simulink model "test_x_eng_sim_packet_4a"  (Simulink 6.2)
settings: Solver=ode45  StartTime=0.0  StopTime=600000  RelTol=1e-3
undefined symbols (not defined in the file or in its folder): ant_bits, BitWidth, cmult_4bit_em
libraries: xbsIndex_r3 x798, casper_library x39, xps_library x27, simulink x1
(part 1 of 6)
settings Model: LastModifiedBy=dsp
settings DebuggingCC: SolverPrmCheckMsg=warning

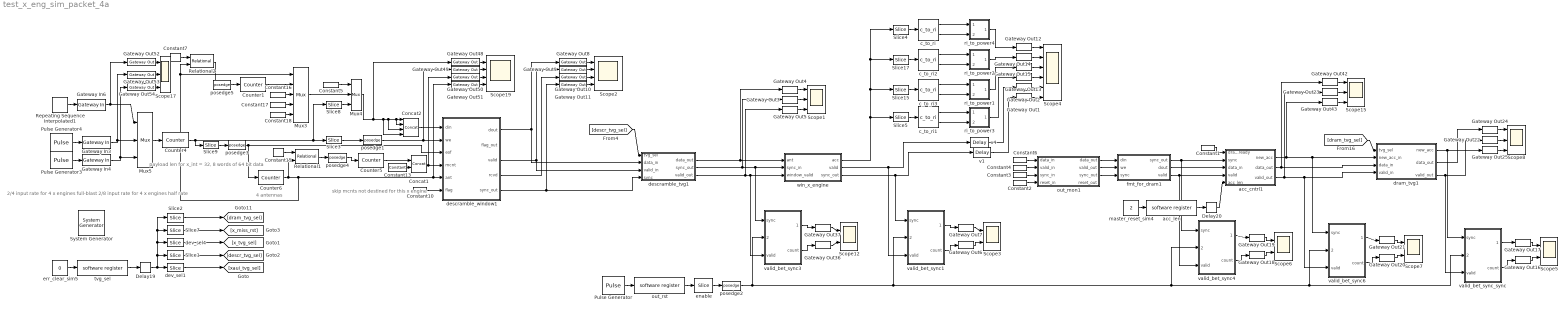
== system test_x_eng_sim_packet_4a ==
  note: 2/4 input rate for 4 x engines full-blast
      | 2/8 input rate for 4 x engines half rate
  note: 4 antennas
  note: skip mcnts not destined
      | for this x engine
  note: payload len
      | for x_int = 32,
      | 8 words of 64 bit data
  " System Generator" : xbsIndex_r3/ System Generator  Tag=genX  xilinxfamily=Virtex2  part=xc2v1000  speed=-4  package=bg575  synthesis_tool=XST  directory=./netlist  testbench=off  simulink_period=1  sysclk_period=100  incr_netlist=off  trim_vbits=Everywhere in SubSystem  dbl_ovrd=According to Block Masks  core_generation=According to Block Masks  run_coregen=off  deprecated_control=off  eval_field=0
      settings: AttributesFormatString=System\nGenerator
  Concat1 : xbsIndex_r3/Concat  num_inputs=2  explicit_period=off  period=1  dbl_ovrd=off
  Concat2 : xbsIndex_r3/Concat  num_inputs=4  explicit_period=off  period=1  dbl_ovrd=off
  Constant1 : xbsIndex_r3/Constant  const=1  equ=P=C  arith_type=Boolean  n_bits=1  bin_pt=0  opselect=C  inp2=PCIN>>17  opr=+  inp1=P  carry=CIN  iostate=0  explicit_period=on  period=1  dbl_ovrd=off
  Constant10 : xbsIndex_r3/Constant  const=0  equ=P=C  arith_type=Unsigned  n_bits=1  bin_pt=0  opselect=C  inp2=PCIN>>17  opr=+  inp1=P  carry=CIN  iostate=0  explicit_period=on  period=1  dbl_ovrd=off
  Constant13 : xbsIndex_r3/Constant  const=0  equ=P=C  arith_type=Unsigned  n_bits=2  bin_pt=0  opselect=C  inp2=PCIN>>17  opr=+  inp1=P  carry=CIN  iostate=0  explicit_period=on  period=1  dbl_ovrd=off
  Constant15 : xbsIndex_r3/Constant  const=0  equ=P=C  arith_type=Unsigned  n_bits=3  bin_pt=0  opselect=C  inp2=PCIN>>17  opr=+  inp1=P  carry=CIN  iostate=0  explicit_period=on  period=1  dbl_ovrd=off
  Constant16 : xbsIndex_r3/Constant  const=0  equ=P=C  arith_type=Unsigned  n_bits=16  bin_pt=0  opselect=C  inp2=PCIN>>17  opr=+  inp1=P  carry=CIN  iostate=0  explicit_period=on  period=1  dbl_ovrd=off
  Constant17 : xbsIndex_r3/Constant  const=0  equ=P=C  arith_type=Unsigned  n_bits=16  bin_pt=0  opselect=C  inp2=PCIN>>17  opr=+  inp1=P  carry=CIN  iostate=0  explicit_period=on  period=1  dbl_ovrd=off
  Constant18 : xbsIndex_r3/Constant  const=0  equ=P=C  arith_type=Unsigned  n_bits=16  bin_pt=0  opselect=C  inp2=PCIN>>17  opr=+  inp1=P  carry=CIN  iostate=0  explicit_period=on  period=1  dbl_ovrd=off
  Constant2 : xbsIndex_r3/Constant  const=0  equ=P=C  arith_type=Boolean  n_bits=1  bin_pt=0  opselect=C  inp2=PCIN>>17  opr=+  inp1=P  carry=CIN  iostate=0  explicit_period=on  period=1  dbl_ovrd=off
  Constant3 : xbsIndex_r3/Constant  const=0  equ=P=C  arith_type=Boolean  n_bits=1  bin_pt=0  opselect=C  inp2=PCIN>>17  opr=+  inp1=P  carry=CIN  iostate=0  explicit_period=on  period=1  dbl_ovrd=off
  Constant4 : xbsIndex_r3/Constant  const=0  equ=P=C  arith_type=Boolean  n_bits=1  bin_pt=0  opselect=C  inp2=PCIN>>17  opr=+  inp1=P  carry=CIN  iostate=0  explicit_period=on  period=1  dbl_ovrd=off
  Constant5 : xbsIndex_r3/Constant  const=0  equ=P=C  arith_type=Unsigned  n_bits=1  bin_pt=0  opselect=C  inp2=PCIN>>17  opr=+  inp1=P  carry=CIN  iostate=0  explicit_period=on  period=1  dbl_ovrd=off
  Constant6 : xbsIndex_r3/Constant  const=0  equ=P=C  arith_type=Unsigned  n_bits=112  bin_pt=0  opselect=C  inp2=PCIN>>17  opr=+  inp1=P  carry=CIN  iostate=0  explicit_period=on  period=1  dbl_ovrd=off
  Constant7 : xbsIndex_r3/Constant  const=0  equ=P=C  arith_type=Unsigned  n_bits=1  bin_pt=0  opselect=C  inp2=PCIN>>17  opr=+  inp1=P  carry=CIN  iostate=0  explicit_period=on  period=1  dbl_ovrd=off
  Counter1 : xbsIndex_r3/Counter  cnt_type=Free Running  n_bits=16  bin_pt=0  arith_type=Unsigned  start_count=0  cnt_to=Inf  cnt_by_val=1  operation=Up  explicit_period=off  period=1  load_pin=off  rst=off  en=on  dbl_ovrd=off  show_param=off  use_rpm=on  gen_core=off
      settings: xl_area=[0, 0, 0, 0, 0, 0, 0]
  Counter4 : xbsIndex_r3/Counter  cnt_type=Free Running  n_bits=32  bin_pt=0  arith_type=Unsigned  start_count=0  cnt_to=32  cnt_by_val=1  operation=Up  explicit_period=off  period=1  load_pin=off  rst=off  en=on  dbl_ovrd=off  show_param=off  use_rpm=on  gen_core=off
      settings: xl_area=[0, 0, 0, 0, 0, 0, 0]
  Counter5 : xbsIndex_r3/Counter  cnt_type=Free Running  n_bits=48-2  bin_pt=0  arith_type=Unsigned  start_count=0  cnt_to=Inf  cnt_by_val=1  operation=Up  explicit_period=off  period=1  load_pin=off  rst=off  en=on  dbl_ovrd=off  show_param=off  use_rpm=on  gen_core=off
      settings: xl_area=[0, 0, 0, 0, 0, 0, 0]
  Counter6 : xbsIndex_r3/Counter  cnt_type=Free Running  n_bits=2  bin_pt=0  arith_type=Unsigned  start_count=0  cnt_to=Inf  cnt_by_val=1  operation=Up  explicit_period=off  period=1  load_pin=off  rst=off  en=on  dbl_ovrd=off  show_param=off  use_rpm=on  gen_core=off
      settings: xl_area=[0, 0, 0, 0, 0, 0, 0]
  Delay19 : xbsIndex_r3/Delay  latency=2  reg_retiming=off  explicit_period=off  period=1  en=off  accept_only_valid=off  init_zero=on  dbl_ovrd=off  show_param=off
      settings: xl_area=[0, 0, 0, 0, 0, 0, 0]
  Delay20 : xbsIndex_r3/Delay  latency=2  reg_retiming=off  explicit_period=off  period=1  en=off  accept_only_valid=off  init_zero=on  dbl_ovrd=off  show_param=off
      settings: xl_area=[0, 0, 0, 0, 0, 0, 0]
  Gateway In3 : xbsIndex_r3/Gateway In  arith_type=Boolean  n_bits=8  bin_pt=6  quantization=Truncate  overflow=Wrap  period=1  timing_constraint=None  locs_specified=off  LOCs={}  needs_fixed_name=off  dbl_ovrd=off  show_param=off
      settings: xl_area=[0, 0, 0, 0, 0, 0, 0]
  Gateway In4 : xbsIndex_r3/Gateway In  arith_type=Boolean  n_bits=8  bin_pt=6  quantization=Truncate  overflow=Wrap  period=1  timing_constraint=None  locs_specified=off  LOCs={}  needs_fixed_name=off  dbl_ovrd=off  show_param=off
      settings: xl_area=[0, 0, 0, 0, 0, 0, 0]
  Gateway In6 : xbsIndex_r3/Gateway In  arith_type=Unsigned  n_bits=1  bin_pt=0  quantization=Truncate  overflow=Wrap  period=1  timing_constraint=None  locs_specified=off  LOCs={}  needs_fixed_name=off  dbl_ovrd=off  show_param=off
      settings: xl_area=[0, 0, 0, 0, 0, 0, 0]
  Gateway Out{1..7,12..25,36..37,42..43} (25 alike) : xbsIndex_r3/Gateway Out  output_type=Double  nbits=8  bin_pt=6  arith_type=Boolean  quantization=Truncate  overflow=Wrap  hdl_port=off  timing_constraint=None  locs_specified=off  LOCs={}  needs_fixed_name=off  show_param=off
      settings: xl_area=[0, 0, 0, 0, 0, 0, 0]
  Gateway Out{8..11,48..54} (11 alike) : xbsIndex_r3/Gateway Out  output_type=Double  nbits=8  bin_pt=6  arith_type=Boolean  quantization=Truncate  overflow=Wrap  hdl_port=on  timing_constraint=None  locs_specified=off  LOCs={}  needs_fixed_name=off  show_param=off
      settings: xl_area=[0, 0, 0, 0, 0, 0, 0]
  Mux3 : xbsIndex_r3/Mux  inputs=4  precision=Full  arith_type="Signed  (2's comp)"  n_bits=8  bin_pt=2  quantization=Truncate  overflow=Wrap  latency=0  explicit_period=off  period=1  en=off  dbl_ovrd=off  show_param=off  mux_type=off  use_rpm=off  gen_core=off
      settings: xl_area=[0, 0, 0, 0, 0, 0, 0]
  Mux4 : xbsIndex_r3/Mux  inputs=2  precision=Full  arith_type="Signed  (2's comp)"  n_bits=8  bin_pt=2  quantization=Truncate  overflow=Wrap  latency=0  explicit_period=off  period=1  en=off  dbl_ovrd=off  show_param=off  mux_type=off  use_rpm=off  gen_core=off
      settings: xl_area=[0, 0, 0, 0, 0, 0, 0]
  Mux5 : xbsIndex_r3/Mux  inputs=2  precision=Full  arith_type="Signed  (2's comp)"  n_bits=8  bin_pt=2  quantization=Truncate  overflow=Wrap  latency=0  explicit_period=off  period=1  en=off  dbl_ovrd=off  show_param=off  mux_type=off  use_rpm=off  gen_core=off
      settings: xl_area=[0, 0, 0, 0, 0, 0, 0]
  Pulse Generator : DiscretePulseGenerator  Period=2^15  PhaseDelay=2^14
  Pulse Generator3 : DiscretePulseGenerator  Period=4  PulseWidth=2
  Pulse Generator4 : DiscretePulseGenerator  PulseWidth=2
  Relational1 : xbsIndex_r3/Relational  mode=a=b  latency=1  explicit_period=off  period=1  en=off  dbl_ovrd=off  show_param=off
      settings: xl_area=[0, 0, 0, 0, 0, 0, 0]
  Relational2 : xbsIndex_r3/Relational  mode=a=b  latency=1  explicit_period=off  period=1  en=off  dbl_ovrd=off  show_param=off
      settings: xl_area=[0, 0, 0, 0, 0, 0, 0]
  Repeating Sequence Interpolated1 : simulink/Sources/Repeating Sequence Interpolated  OutValues=[0 1].'  TimeValues=[100000 300000].'  LookUpMeth=Use Input Above  tsamp=1  OutputDataTypeScalingMode=Specify via dialog  OutDataType=float('double')  OutScaling=2^-10
  Scope{1,8,15,17} (4 alike) : Scope  NumInputPorts=3
      Scope1 settings: YMin=-1~-1~-5  YMax=1~1~5  SaveName=ScopeData5
      Scope15 settings: YMin=0~0~-1  YMax=1.4e+011~1~1  SaveName=ScopeData12
      Scope17 settings: YMin=-1~0~0  YMax=1~1~1  SaveName=ScopeData9
      Scope8 settings: YMin=0~0~-1  YMax=1.1e+011~1~1  SaveName=ScopeData10
  Scope{3,5..7,12} (5 alike) : Scope  NumInputPorts=2
      Scope12 settings: YMin=31128.7~9840  YMax=34405.3~10060  SaveName=data_into_xeng
      Scope3 settings: YMin=2560~1140  YMax=2560~1150  SaveName=data_into_xeng1
      Scope5 settings: YMin=9727.05~819  YMax=10751~839  SaveName=ScopeData6
      Scope6 settings: YMin=4864~2340  YMax=5376~2360  SaveName=ScopeData4
      Scope7 settings: YMin=0~0  YMax=10500~10500  SaveName=ScopeData8
  Scope19 : Scope  NumInputPorts=4
      settings: YMin=0~0~28~0  YMax=1~1~40~3  SaveName=ScopeData14
  Scope2 : Scope  NumInputPorts=4
      settings: YMin=0~1~1~0  YMax=32.5~1~1~1
  Scope4 : Scope  NumInputPorts=6
      settings: YMin=-1~0~-1~-1~0~-1  YMax=1~4~1~1~1~1  SaveName=ScopeData7
  Slice1 : xbsIndex_r3/Slice  mode=Lower Bit Location + Width  nbits=2  bit1=0  base1=MSB of Input  bit0=1  base0=LSB of Input  boolean_output=on  explicit_period=off  period=1  dbl_ovrd=off
  Slice15 : xbsIndex_r3/Slice  mode=Lower Bit Location + Width  nbits=112/4  bit1=0  base1=MSB of Input  bit0=112/4  base0=LSB of Input  boolean_output=off  explicit_period=off  period=1  dbl_ovrd=off
  Slice17 : xbsIndex_r3/Slice  mode=Lower Bit Location + Width  nbits=112/4  bit1=0  base1=MSB of Input  bit0=112/4*2  base0=LSB of Input  boolean_output=off  explicit_period=off  period=1  dbl_ovrd=off
  Slice2 : xbsIndex_r3/Slice  mode=Lower Bit Location + Width  nbits=5  bit1=0  base1=MSB of Input  bit0=9  base0=LSB of Input  boolean_output=off  explicit_period=off  period=1  dbl_ovrd=off
  Slice3 : xbsIndex_r3/Slice  mode=Lower Bit Location + Width  nbits=1  bit1=0  base1=MSB of Input  bit0=0  base0=LSB of Input  boolean_output=on  explicit_period=off  period=1  dbl_ovrd=off
  Slice4 : xbsIndex_r3/Slice  mode=Lower Bit Location + Width  nbits=112/4  bit1=0  base1=MSB of Input  bit0=112/4*3  base0=LSB of Input  boolean_output=off  explicit_period=off  period=1  dbl_ovrd=off
  Slice5 : xbsIndex_r3/Slice  mode=Lower Bit Location + Width  nbits=112/4  bit1=0  base1=MSB of Input  bit0=0  base0=LSB of Input  boolean_output=off  explicit_period=off  period=1  dbl_ovrd=off
  Slice7 : xbsIndex_r3/Slice  mode=Lower Bit Location + Width  nbits=1  bit1=0  base1=MSB of Input  bit0=8  base0=LSB of Input  boolean_output=on  explicit_period=off  period=1  dbl_ovrd=off
  Slice8 : xbsIndex_r3/Slice  mode=Lower Bit Location + Width  nbits=16  bit1=0  base1=MSB of Input  bit0=1  base0=LSB of Input  boolean_output=on  explicit_period=off  period=1  dbl_ovrd=off
  Slice9 : xbsIndex_r3/Slice  mode=Lower Bit Location + Width  nbits=1  bit1=0  base1=MSB of Input  bit0=4  base0=LSB of Input  boolean_output=on  explicit_period=off  period=1  dbl_ovrd=off
  acc_cntrl1 : Subsystem
  acc_len : xps_library/software register  Tag=xps:sw_reg  io_dir=From Processor  arith_type=Unsigned  bitwidth=32  bin_pt=0  sample_period=1  gw_name=test_x_eng_sim_packet_4a_acc_len_user_data_out
  c_to_ri{,1..3} (4 alike) : casper_library/Misc/c_to_ri  n_bits=16  bin_pt=6
      settings: AttributesFormatString=16_6 r/i
  descramble_tvg1 : Subsystem  mask{ant_bits=2, x_int_bits=5, sync_period=15}
      mask prompts: ant_bits "Number of Antennas (2^?):"; x_int_bits "X Integration Length (2^?):"; sync_period "Sync Pulse Period (2^?):"
  descramble_window1 : Subsystem  mask{ant_bits=2, x_int_bits=5, window_bits=3, sync_bits=11}
      mask prompts: ant_bits "Maximum Number of Antennas (2^?):"; x_int_bits "X Engine Integration Length (2^?):"; window_bits "Number of Windows to Buffer (2^?):"; sync_bits "Samples Between Sync Pulses (2^?)"
      mask help: Valids between sync pulses: Would like this to come after every dram_vecc_len: valids_bet_syncs = xeng_int_len * num_ants * freqs_per_xeng. Normally, num_ants = num_xeng so this simplifies to xeng_int_len * n_chans.
  dev_sel1 : xbsIndex_r3/Slice  mode=Lower Bit Location + Width  nbits=1  bit1=0  base1=MSB of Input  bit0=0  base0=LSB of Input  boolean_output=off  explicit_period=off  period=1  dbl_ovrd=off
  dev_sel4 : xbsIndex_r3/Slice  mode=Lower Bit Location + Width  nbits=2  bit1=0  base1=MSB of Input  bit0=3  base0=LSB of Input  boolean_output=off  explicit_period=off  period=1  dbl_ovrd=off
  dram_tvg1 : Subsystem  mask{len=18432}
      mask prompts: len "Number of Vectors"
  enable : xbsIndex_r3/Slice  mode=Lower Bit Location + Width  nbits=1  bit1=0  base1=LSB of Input  bit0=0  base0=LSB of Input  boolean_output=on  explicit_period=off  period=1  dbl_ovrd=off
  err_clear_sim5 : Constant  Value=0
  fmt_for_dram1 : Subsystem  mask{x_int_bits=5, x_n_bits=4}
      mask prompts: x_int_bits "X Engine integration length (2^?):"; x_n_bits "X Engine input bits"
  master_reset_sim4 : Constant  Value=2
  out_mon1 : Subsystem  mask{n_ants=4, n_chans=512}
      mask prompts: n_ants "Number of Antennas"; n_chans "Number of Frequency Channels in the system"
  out_rst : xps_library/software register  Tag=xps:sw_reg  io_dir=From Processor  arith_type=Unsigned  bitwidth=32  bin_pt=0  sample_period=1  gw_name=test_x_eng_sim_packet_4a_out_rst_user_data_out
  posedge{1..5} (5 alike) : casper_library/Misc/posedge  Tag=Rising Edge Detector
  ri_to_power1 : Subsystem
  ri_to_power2 : Subsystem
  ri_to_power3 : Subsystem
  ri_to_power4 : Subsystem
  tvg_sel : xps_library/software register  Tag=xps:sw_reg  io_dir=From Processor  arith_type=Unsigned  bitwidth=32  bin_pt=0  sample_period=1  gw_name=test_x_eng_sim_packet_4a_tvg_sel_user_data_out
  v1 : xbsIndex_r3/Delay  latency=5  reg_retiming=off  explicit_period=off  period=1  en=off  accept_only_valid=off  init_zero=on  dbl_ovrd=off  show_param=off
      settings: xl_area=[0, 0, 0, 0, 0, 0, 0]
  v4 : xbsIndex_r3/Delay  latency=5  reg_retiming=off  explicit_period=off  period=1  en=off  accept_only_valid=off  init_zero=on  dbl_ovrd=off  show_param=off
      settings: xl_area=[0, 0, 0, 0, 0, 0, 0]
  valid_bet_sync1 : Subsystem
  valid_bet_sync3 : Subsystem
  valid_bet_sync4 : Subsystem
  valid_bet_sync6 : Subsystem
  valid_bet_sync_sync : Subsystem
  win_x_engine : Subsystem  AncestorBlock=casper_library/Correlator/x_engine  mask(x_engine){n_ants=4, n_bits=4, acc_len=32, add_latency=1, mult_latency=1, bram_latency=1, use_ded_mult=1, use_bram_delay=1}
      mask prompts: n_ants "Number of Antennas"; n_bits "Bit Width of Samples In"; acc_len "Accumulation Length"; add_latency "Add Latency"; mult_latency "Mult Latency"; bram_latency "BRAM Latency"; use_ded_mult "Multiplier Type (0=slices 1=embedded 2=bram)"; use_bram_delay "Delay in BRAM"
      mask init:
      | bit_growth = ceil(log2(acc_len));
      | ant_bits = ceil(log2(n_ants));
      | n_bits_out = (2*n_bits + 1 + bit_growth);
      | 
      | win_x_engine_init(gcb, ...
      |     'n_ants', n_ants, ...
      |     'n_bits', n_bits, ...
      |     'acc_len', acc_len, ...
      |     'add_latency', add_latency, ...
      |     'mult_latency', mult_latency, ...
      |     'bram_latency', bram_latency, ...
      |     'use_ded_mult', use_ded_mult, ...
      |     'use_bram_delay', use_bram_delay);
      settings: AttributesFormatString=n_ant=4, bits=4, mult=1, bram=1
  wires:
  [descr_tvg_sel] -> descramble_tvg1/1(tvg_sel)
  descramble_tvg1/1(data_out) -> win_x_engine/1(ant), Gateway Out4/1
  out_rst/1 -> enable/1
  Pulse Generator/1 -> out_rst/1
  enable/1 -> posedge2/1
  posedge2/1 -> valid_bet_sync3/2(rst_max), valid_bet_sync1/2(rst_max), valid_bet_sync4/2(rst_max), valid_bet_sync6/2(rst_max), valid_bet_sync_sync/2(rst_max)
  Gateway Out8/1 -> Scope2/1
  Gateway Out9/1 -> Scope2/2
  Gateway Out10/1 -> Scope2/3
  Gateway Out11/1 -> Scope2/4
  err_clear_sim5/1 -> tvg_sel/1
  tvg_sel/1 -> Delay19/1
  Delay19/1 -> dev_sel1/1, Slice1/1, dev_sel4/1, Slice2/1, Slice7/1
  dev_sel1/1 -> [xaui_tvg_sel]
  Slice1/1 -> [descr_tvg_sel]
  dev_sel4/1 -> [x_tvg_sel]
  Slice7/1 -> [x_miss_rst]
  Slice2/1 -> [dram_tvg_sel]
  Gateway Out36/1 -> Scope12/2
  Gateway Out37/1 -> Scope12/1
  valid_bet_sync3/1(max_count) -> Gateway Out37/1
  valid_bet_sync3/2(count) -> Gateway Out36/1
  Constant10/1 -> descramble_window1/6(flag)
  Gateway Out48/1 -> Scope19/1
  Gateway Out49/1 -> Scope19/2
  Gateway Out50/1 -> Scope19/3
  Gateway Out51/1 -> Scope19/4
  Constant13/1 -> Concat1/2
  Concat1/1 -> Gateway Out50/1, descramble_window1/4(mcnt)
  Counter5/1 -> Concat1/1
  Counter6/1 -> Relational1/2, Gateway Out51/1, descramble_window1/5(ant), Mux3/1, Relational2/2
  Concat2/1 -> descramble_window1/1(din)
  Relational1/1 -> posedge4/1
  Constant15/1 -> Relational1/1
  Slice3/1 -> posedge1/1
  Counter4/1 -> Slice9/1, Slice3/1, Slice8/1
  Mux4/1 -> Concat2/4, Concat2/3, Concat2/1, Concat2/2, Gateway Out48/1
  Slice9/1 -> posedge3/1
  posedge3/1 -> Counter6/1, descramble_window1/3(eof)
  posedge4/1 -> Counter5/1
  Pulse Generator3/1 -> Gateway In4/1
  Counter1/1 -> Mux3/2
  Constant16/1 -> Mux3/3
  Constant17/1 -> Mux3/4
  Constant18/1 -> Mux3/5
  Mux3/1 -> Mux4/2
  Slice8/1 -> Mux4/3
  Constant5/1 -> Mux4/1
  Pulse Generator4/1 -> Gateway In3/1
  Mux5/1 -> Counter4/1
  Gateway In3/1 -> Gateway Out53/1, Mux5/2
  Gateway In4/1 -> Gateway Out54/1, Mux5/3
  Gateway In6/1 -> Mux5/1, Gateway Out52/1
  Repeating Sequence Interpolated1/1 -> Gateway In6/1
  Gateway Out52/1 -> Scope17/1
  Gateway Out53/1 -> Scope17/2
  Gateway Out54/1 -> Scope17/3
  descramble_tvg1/3(valid_out) -> valid_bet_sync3/3(valid), win_x_engine/3(window_valid), Gateway Out5/1
  posedge1/1 -> Gateway Out49/1, descramble_window1/2(we)
  win_x_engine/1(acc) -> Slice4/1, Slice17/1, Slice15/1, Slice5/1
  win_x_engine/2(valid) -> valid_bet_sync1/3(valid), v4/1
  win_x_engine/3(sync_out) -> valid_bet_sync1/1(sync), v1/1
  descramble_tvg1/2(sync_out) -> valid_bet_sync3/1(sync), win_x_engine/2(sync_in), Gateway Out3/1
  Slice4/1 -> c_to_ri/1
  Slice17/1 -> c_to_ri2/1
  Slice15/1 -> c_to_ri3/1
  Slice5/1 -> c_to_ri1/1
  c_to_ri/1 -> ri_to_power4/1(In1)
  c_to_ri/2 -> ri_to_power4/2(In2)
  c_to_ri2/1 -> ri_to_power2/1(In1)
  c_to_ri2/2 -> ri_to_power2/2(In2)
  c_to_ri3/1 -> ri_to_power1/1(In1)
  c_to_ri3/2 -> ri_to_power1/2(In2)
  c_to_ri1/1 -> ri_to_power3/1(In1)
  c_to_ri1/2 -> ri_to_power3/2(In2)
  Gateway Out15/1 -> Scope4/3
  Gateway Out14/1 -> Scope4/2
  Gateway Out12/1 -> Scope4/1
  Gateway Out13/1 -> Scope4/4
  ri_to_power4/1(Out1) -> Gateway Out12/1
  ri_to_power2/1(Out1) -> Gateway Out14/1
  ri_to_power1/1(Out1) -> Gateway Out15/1
  ri_to_power3/1(Out1) -> Gateway Out13/1
  Gateway Out2/1 -> Scope4/5
  Gateway Out1/1 -> Scope4/6
  Gateway Out3/1 -> Scope1/2
  Gateway Out4/1 -> Scope1/1
  Gateway Out5/1 -> Scope1/3
  Gateway Out6/1 -> Scope3/2
  Gateway Out7/1 -> Scope3/1
  valid_bet_sync1/1(max_count) -> Gateway Out7/1
  valid_bet_sync1/2(count) -> Gateway Out6/1
  v1/1 -> Gateway Out1/1
  v4/1 -> Gateway Out2/1
  out_mon1/3(sync_out) -> fmt_for_dram1/3(sync)
  out_mon1/2(valid_out) -> fmt_for_dram1/2(we)
  out_mon1/1(data_out) -> fmt_for_dram1/1(din)
  acc_len/1 -> Delay20/1
  master_reset_sim4/1 -> acc_len/1
  fmt_for_dram1/1(sync_out) -> valid_bet_sync4/1(sync), acc_cntrl1/2(sync)
  fmt_for_dram1/2(dout) -> acc_cntrl1/3(data_in)
  fmt_for_dram1/3(valid) -> valid_bet_sync4/3(valid), acc_cntrl1/4("valid ")
  acc_cntrl1/1(new_acc) -> Gateway Out43/1, valid_bet_sync6/1(sync), dram_tvg1/2(new_acc_in)
  acc_cntrl1/3(valid_out) -> Gateway Out23/1, valid_bet_sync6/3(valid), dram_tvg1/4(valid_in)
  Delay20/1 -> acc_cntrl1/5(acc_len)
  Constant1/1 -> acc_cntrl1/1(dram_ready)
  Gateway Out18/1 -> Scope6/2
  Gateway Out19/1 -> Scope6/1
  valid_bet_sync4/1(max_count) -> Gateway Out19/1
  valid_bet_sync4/2(count) -> Gateway Out18/1
  Gateway Out20/1 -> Scope7/2
  Gateway Out21/1 -> Scope7/1
  valid_bet_sync6/1(max_count) -> Gateway Out21/1
  valid_bet_sync6/2(count) -> Gateway Out20/1
  Gateway Out23/1 -> Scope15/2
  Gateway Out42/1 -> Scope15/1
  Gateway Out43/1 -> Scope15/3
  acc_cntrl1/2(data_out) -> Gateway Out42/1, dram_tvg1/3(data_in)
  [dram_tvg_sel] -> dram_tvg1/1(tvg_sel)
  Gateway Out16/1 -> Scope5/2
  Gateway Out17/1 -> Scope5/1
  valid_bet_sync_sync/1(max_count) -> Gateway Out17/1
  valid_bet_sync_sync/2(count) -> Gateway Out16/1
  dram_tvg1/3(valid_out) -> Gateway Out22/1, valid_bet_sync_sync/3(valid)
  dram_tvg1/1(new_acc) -> Gateway Out25/1, valid_bet_sync_sync/1(sync)
  Gateway Out22/1 -> Scope8/2
  Gateway Out24/1 -> Scope8/1
  Gateway Out25/1 -> Scope8/3
  dram_tvg1/2(data_out) -> Gateway Out24/1
  Constant6/1 -> out_mon1/1(data_in)
  Constant4/1 -> out_mon1/2(valid_in)
  Constant3/1 -> out_mon1/3(sync_in)
  Constant2/1 -> out_mon1/4(reset_in)
  descramble_window1/1(dout) -> descramble_tvg1/2(data_in), Gateway Out8/1
  descramble_window1/3(valid) -> descramble_tvg1/3(valid_in), Gateway Out9/1
  descramble_window1/5(sync_out) -> descramble_tvg1/4(sync), Gateway Out11/1
  descramble_window1/4(rcvd) -> Gateway Out10/1
  Relational2/1 -> posedge5/1
  Constant7/1 -> Relational2/1
  posedge5/1 -> Counter1/1

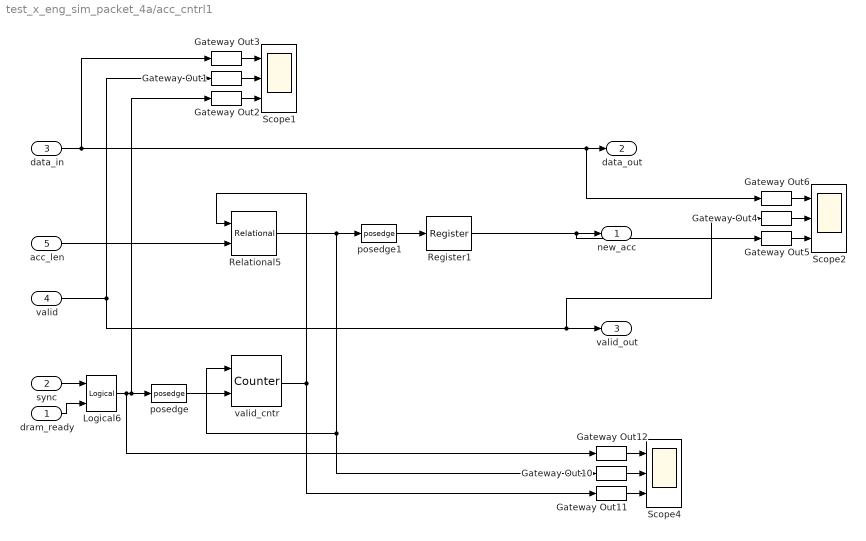
== system test_x_eng_sim_packet_4a/acc_cntrl1 ==
  dram_ready : Inport  Port=1  LatchInput=off
  sync : Inport  Port=2  LatchInput=off
  data_in : Inport  Port=3  LatchInput=off
  "valid " : Inport  Port=4  LatchInput=off
  acc_len : Inport  Port=5  LatchInput=off
  Gateway Out{1..6,10..12} (9 alike) : xbsIndex_r3/Gateway Out  output_type=Double  nbits=8  bin_pt=6  arith_type=Boolean  quantization=Truncate  overflow=Wrap  hdl_port=off  timing_constraint=None  locs_specified=off  LOCs={}  needs_fixed_name=off  show_param=off
      settings: xl_area=[0, 0, 0, 0, 0, 0, 0]
  Logical6 : xbsIndex_r3/Logical  logical_function=AND  inputs=2  precision=Full  arith_type=Unsigned  n_bits=8  bin_pt=2  align_bp=on  latency=0  explicit_period=off  period=1  en=off  dbl_ovrd=off  show_param=off
      settings: xl_area=[0, 0, 0, 0, 0, 0, 0]
  Register1 : xbsIndex_r3/Register  init=0  reg_only_valid=off  explicit_period=off  period=1  rst=off  en=off  out_en=off  dbl_ovrd=off  show_param=off
      settings: xl_area=[0, 0, 0, 0, 0, 0, 0]
  Relational5 : xbsIndex_r3/Relational  mode=a=b  latency=0  explicit_period=on  period=1  en=off  dbl_ovrd=off  show_param=off
      settings: xl_area=[0, 0, 0, 0, 0, 0, 0]
  Scope1 : Scope  NumInputPorts=3
      settings: YMin=2.15512e+037~-1~-1  YMax=2.38198e+037~1~1  SaveName=ScopeData2
  Scope2 : Scope  NumInputPorts=3
      settings: YMin=0~1~0  YMax=3e+011~1~1  SaveName=ScopeData3
  Scope4 : Scope  NumInputPorts=3
      settings: YMin=2.15512e+037~-1~-1  YMax=2.38198e+037~1~1
  posedge : casper_library/Misc/posedge  Tag=Rising Edge Detector
  posedge1 : casper_library/Misc/posedge  Tag=Rising Edge Detector
  valid_cntr : xbsIndex_r3/Counter  cnt_type=Free Running  n_bits=32  bin_pt=0  arith_type=Unsigned  start_count=0  cnt_to=Inf  cnt_by_val=1  operation=Up  explicit_period=on  period=1  load_pin=off  rst=on  en=on  dbl_ovrd=off  show_param=off  use_rpm=on  gen_core=off
      settings: xl_area=[0, 0, 0, 0, 0, 0, 0]
  new_acc : Outport
  data_out : Outport  Port=2
  valid_out : Outport  Port=3
  wires:
  "valid "/1 -> Gateway Out1/1, valid_out/1, Gateway Out4/1
  sync/1 -> Logical6/1
  dram_ready/1 -> Logical6/2
  Logical6/1 -> Gateway Out12/1, posedge/1, Gateway Out2/1
  posedge/1 -> valid_cntr/2
  Relational5/1 -> posedge1/1, Gateway Out10/1, valid_cntr/1
  valid_cntr/1 -> Relational5/1, Gateway Out11/1
  acc_len/1 -> Relational5/2
  data_in/1 -> Gateway Out3/1, data_out/1, Gateway Out6/1
  Gateway Out11/1 -> Scope4/3
  Gateway Out10/1 -> Scope4/2
  Gateway Out12/1 -> Scope4/1
  Gateway Out2/1 -> Scope1/3
  Gateway Out1/1 -> Scope1/2
  Gateway Out3/1 -> Scope1/1
  Gateway Out5/1 -> Scope2/3
  Gateway Out4/1 -> Scope2/2
  Gateway Out6/1 -> Scope2/1
  posedge1/1 -> Register1/1
  Register1/1 -> new_acc/1, Gateway Out5/1

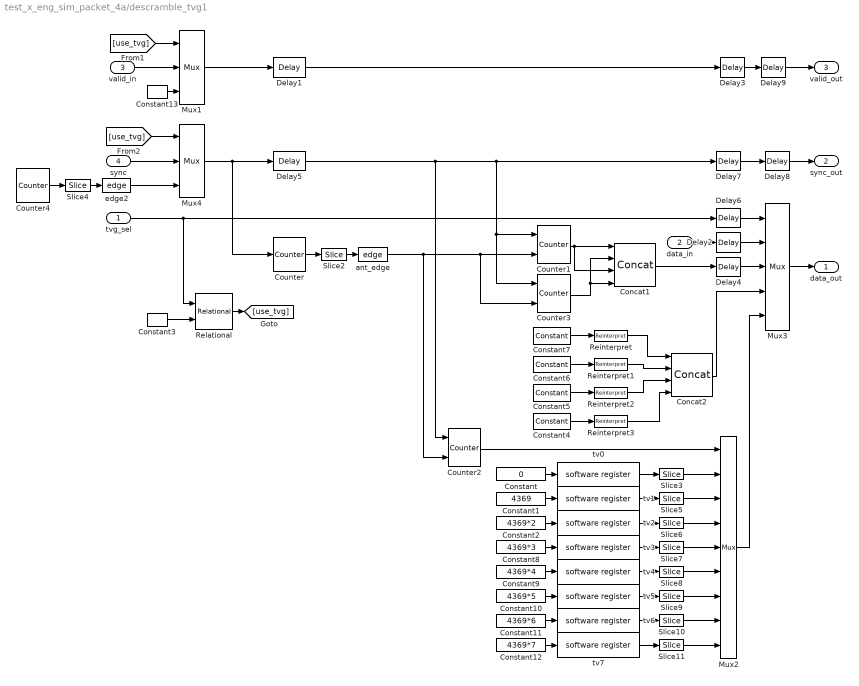
== system test_x_eng_sim_packet_4a/descramble_tvg1 ==
  tvg_sel : Inport  Port=1  LatchInput=off
  data_in : Inport  Port=2  LatchInput=off
  valid_in : Inport  Port=3  LatchInput=off
  sync : Inport  Port=4  LatchInput=off
  Concat1 : xbsIndex_r3/Concat  num_inputs=4  explicit_period=off  period=1  dbl_ovrd=off
  Concat2 : xbsIndex_r3/Concat  num_inputs=4  explicit_period=off  period=1  dbl_ovrd=off
  Constant : Constant  Value=0
  Constant1 : Constant  Value=4369
  Constant10 : Constant  Value=4369*5
  Constant11 : Constant  Value=4369*6
  Constant12 : Constant  Value=4369*7
  Constant13 : xbsIndex_r3/Constant  const=1  equ=P=C  arith_type=Boolean  n_bits=1  bin_pt=0  opselect=C  inp2=PCIN>>17  opr=+  inp1=P  carry=CIN  iostate=0  explicit_period=on  period=1  dbl_ovrd=off
  Constant2 : Constant  Value=4369*2
  Constant3 : xbsIndex_r3/Constant  const=0  equ=P=C  arith_type=Unsigned  n_bits=2  bin_pt=0  opselect=C  inp2=PCIN>>17  opr=+  inp1=P  carry=CIN  iostate=0  explicit_period=on  period=1  dbl_ovrd=off
  Constant4 : xbsIndex_r3/Constant  const=-0.25  equ=P=C  arith_type="Signed  (2's comp)"  n_bits=4  bin_pt=3  opselect=C  inp2=PCIN>>17  opr=+  inp1=P  carry=CIN  iostate=0  explicit_period=on  period=1  dbl_ovrd=off
  Constant5 : xbsIndex_r3/Constant  const=0.5  equ=P=C  arith_type="Signed  (2's comp)"  n_bits=4  bin_pt=3  opselect=C  inp2=PCIN>>17  opr=+  inp1=P  carry=CIN  iostate=0  explicit_period=on  period=1  dbl_ovrd=off
  Constant6 : xbsIndex_r3/Constant  const=-6/8  equ=P=C  arith_type="Signed  (2's comp)"  n_bits=4  bin_pt=3  opselect=C  inp2=PCIN>>17  opr=+  inp1=P  carry=CIN  iostate=0  explicit_period=on  period=1  dbl_ovrd=off
  Constant7 : xbsIndex_r3/Constant  const=0.1  equ=P=C  arith_type="Signed  (2's comp)"  n_bits=4  bin_pt=3  opselect=C  inp2=PCIN>>17  opr=+  inp1=P  carry=CIN  iostate=0  explicit_period=on  period=1  dbl_ovrd=off
  Constant8 : Constant  Value=4369*3
  Constant9 : Constant  Value=4369*4
  Counter : xbsIndex_r3/Counter  cnt_type=Free Running  n_bits=x_int_bits + 1  bin_pt=0  arith_type=Unsigned  start_count=0  cnt_to=Inf  cnt_by_val=1  operation=Up  explicit_period=off  period=1  load_pin=off  rst=on  en=off  dbl_ovrd=off  show_param=off  use_rpm=on  gen_core=off
      settings: xl_area=[0, 0, 0, 0, 0, 0, 0]
  Counter1 : xbsIndex_r3/Counter  cnt_type=Free Running  n_bits=4  bin_pt=0  arith_type=Unsigned  start_count=0  cnt_to=7  cnt_by_val=1  operation=Up  explicit_period=off  period=1  load_pin=off  rst=on  en=on  dbl_ovrd=off  show_param=off  use_rpm=on  gen_core=off
      settings: xl_area=[0, 0, 0, 0, 0, 0, 0]
  Counter2 : xbsIndex_r3/Counter  cnt_type=Free Running  n_bits=3  bin_pt=0  arith_type=Unsigned  start_count=0  cnt_to=7  cnt_by_val=1  operation=Up  explicit_period=off  period=1  load_pin=off  rst=on  en=on  dbl_ovrd=off  show_param=off  use_rpm=on  gen_core=off
      settings: xl_area=[0, 0, 0, 0, 0, 0, 0]
  Counter3 : xbsIndex_r3/Counter  cnt_type=Free Running  n_bits=4  bin_pt=0  arith_type=Unsigned  start_count=15  cnt_to=0  cnt_by_val=1  operation=Down  explicit_period=off  period=1  load_pin=off  rst=on  en=on  dbl_ovrd=off  show_param=off  use_rpm=on  gen_core=off
      settings: xl_area=[0, 0, 0, 0, 0, 0, 0]
  Counter4 : xbsIndex_r3/Counter  cnt_type=Free Running  n_bits=sync_period+1  bin_pt=0  arith_type=Unsigned  start_count=2^sync_period - 2  cnt_to=Inf  cnt_by_val=1  operation=Up  explicit_period=off  period=1  load_pin=off  rst=off  en=off  dbl_ovrd=off  show_param=off  use_rpm=on  gen_core=off
      settings: xl_area=[0, 0, 0, 0, 0, 0, 0]
  Delay{1,3..9} (8 alike) : xbsIndex_r3/Delay  latency=1  reg_retiming=off  explicit_period=off  period=1  en=off  accept_only_valid=off  init_zero=on  dbl_ovrd=off  show_param=off
      settings: xl_area=[0, 0, 0, 0, 0, 0, 0]
  Delay2 : xbsIndex_r3/Delay  latency=2  reg_retiming=off  explicit_period=off  period=1  en=off  accept_only_valid=off  init_zero=on  dbl_ovrd=off  show_param=off
      settings: xl_area=[0, 0, 0, 0, 0, 0, 0]
  Mux1 : xbsIndex_r3/Mux  inputs=2  precision=Full  arith_type="Signed  (2's comp)"  n_bits=8  bin_pt=2  quantization=Truncate  overflow=Wrap  latency=0  explicit_period=on  period=1  en=off  dbl_ovrd=off  show_param=off  mux_type=off  use_rpm=off  gen_core=off
      settings: xl_area=[0, 0, 0, 0, 0, 0, 0]
  Mux2 : xbsIndex_r3/Mux  inputs=8  precision=Full  arith_type="Signed  (2's comp)"  n_bits=8  bin_pt=2  quantization=Truncate  overflow=Wrap  latency=1  explicit_period=off  period=1  en=off  dbl_ovrd=off  show_param=off  mux_type=off  use_rpm=off  gen_core=off
      settings: xl_area=[0, 0, 0, 0, 0, 0, 0]
  Mux3 : xbsIndex_r3/Mux  inputs=4  precision=Full  arith_type="Signed  (2's comp)"  n_bits=8  bin_pt=2  quantization=Truncate  overflow=Wrap  latency=1  explicit_period=off  period=1  en=off  dbl_ovrd=off  show_param=off  mux_type=off  use_rpm=off  gen_core=off
      settings: xl_area=[0, 0, 0, 0, 0, 0, 0]
  Mux4 : xbsIndex_r3/Mux  inputs=2  precision=Full  arith_type="Signed  (2's comp)"  n_bits=8  bin_pt=2  quantization=Truncate  overflow=Wrap  latency=0  explicit_period=on  period=1  en=off  dbl_ovrd=off  show_param=off  mux_type=off  use_rpm=off  gen_core=off
      settings: xl_area=[0, 0, 0, 0, 0, 0, 0]
  Reinterpret{,1..3} (4 alike) : xbsIndex_r3/Reinterpret  force_arith_type=on  arith_type=Unsigned  force_bin_pt=on  bin_pt=0  force_valid=on
  Relational : xbsIndex_r3/Relational  mode=a!=b  latency=1  explicit_period=off  period=1  en=off  dbl_ovrd=off  show_param=off
      settings: xl_area=[0, 0, 0, 0, 0, 0, 0]
  Slice{3,5..11} (8 alike) : xbsIndex_r3/Slice  mode=Lower Bit Location + Width  nbits=16  bit1=0  base1=MSB of Input  bit0=0  base0=LSB of Input  boolean_output=off  explicit_period=off  period=1  dbl_ovrd=off
  Slice2 : xbsIndex_r3/Slice  mode=Lower Bit Location + Width  nbits=1  bit1=0  base1=MSB of Input  bit0=x_int_bits  base0=LSB of Input  boolean_output=on  explicit_period=off  period=1  dbl_ovrd=off
  Slice4 : xbsIndex_r3/Slice  mode=Lower Bit Location + Width  nbits=1  bit1=0  base1=MSB of Input  bit0=sync_period  base0=LSB of Input  boolean_output=on  explicit_period=off  period=1  dbl_ovrd=off
  ant_edge : casper_library/Misc/edge
  edge2 : casper_library/Misc/edge
  tv0 : xps_library/software register  Tag=xps:sw_reg  io_dir=From Processor  arith_type=Unsigned  bitwidth=32  bin_pt=0  sample_period=1  gw_name=test_x_eng_sim_packet_4a_descramble_tvg1_tv0_user_data_out
  tv1 : xps_library/software register  Tag=xps:sw_reg  io_dir=From Processor  arith_type=Unsigned  bitwidth=32  bin_pt=0  sample_period=1  gw_name=test_x_eng_sim_packet_4a_descramble_tvg1_tv1_user_data_out
  tv2 : xps_library/software register  Tag=xps:sw_reg  io_dir=From Processor  arith_type=Unsigned  bitwidth=32  bin_pt=0  sample_period=1  gw_name=test_x_eng_sim_packet_4a_descramble_tvg1_tv2_user_data_out
  tv3 : xps_library/software register  Tag=xps:sw_reg  io_dir=From Processor  arith_type=Unsigned  bitwidth=32  bin_pt=0  sample_period=1  gw_name=test_x_eng_sim_packet_4a_descramble_tvg1_tv3_user_data_out
  tv4 : xps_library/software register  Tag=xps:sw_reg  io_dir=From Processor  arith_type=Unsigned  bitwidth=32  bin_pt=0  sample_period=1  gw_name=test_x_eng_sim_packet_4a_descramble_tvg1_tv4_user_data_out
  tv5 : xps_library/software register  Tag=xps:sw_reg  io_dir=From Processor  arith_type=Unsigned  bitwidth=32  bin_pt=0  sample_period=1  gw_name=test_x_eng_sim_packet_4a_descramble_tvg1_tv5_user_data_out
  tv6 : xps_library/software register  Tag=xps:sw_reg  io_dir=From Processor  arith_type=Unsigned  bitwidth=32  bin_pt=0  sample_period=1  gw_name=test_x_eng_sim_packet_4a_descramble_tvg1_tv6_user_data_out
  tv7 : xps_library/software register  Tag=xps:sw_reg  io_dir=From Processor  arith_type=Unsigned  bitwidth=32  bin_pt=0  sample_period=1  gw_name=test_x_eng_sim_packet_4a_descramble_tvg1_tv7_user_data_out
  data_out : Outport
  sync_out : Outport  Port=2
  valid_out : Outport  Port=3
  wires:
  Counter1/1 -> Concat1/1, Concat1/3
  ant_edge/1 -> Counter2/2, Counter1/2, Counter3/2
  Counter/1 -> Slice2/1
  Slice2/1 -> ant_edge/1
  Concat1/1 -> Delay4/1
  Delay8/1 -> sync_out/1
  data_in/1 -> Delay2/1
  Delay2/1 -> Mux3/2
  Mux3/1 -> data_out/1
  Delay3/1 -> Delay9/1
  tvg_sel/1 -> Delay6/1, Relational/1
  Delay6/1 -> Mux3/1
  Constant3/1 -> Relational/2
  Concat2/1 -> Mux3/4
  Counter3/1 -> Concat1/2, Concat1/4
  Delay7/1 -> Delay8/1
  Delay5/1 -> Delay7/1, Counter1/1, Counter3/1, Counter2/1
  Delay4/1 -> Mux3/3
  Relational/1 -> [use_tvg]
  [use_tvg] -> Mux4/1
  Slice4/1 -> edge2/1
  Counter4/1 -> Slice4/1
  sync/1 -> Mux4/2
  Mux4/1 -> Delay5/1, Counter/1
  tv0/1 -> Slice3/1
  Constant/1 -> tv0/1
  Mux2/1 -> Mux3/5
  Slice3/1 -> Mux2/2
  Counter2/1 -> Mux2/1
  tv1/1 -> Slice5/1
  tv2/1 -> Slice6/1
  tv3/1 -> Slice7/1
  tv4/1 -> Slice8/1
  tv5/1 -> Slice9/1
  tv6/1 -> Slice10/1
  tv7/1 -> Slice11/1
  Slice5/1 -> Mux2/3
  Slice6/1 -> Mux2/4
  Slice7/1 -> Mux2/5
  Slice8/1 -> Mux2/6
  Slice9/1 -> Mux2/7
  Slice10/1 -> Mux2/8
  Slice11/1 -> Mux2/9
  edge2/1 -> Mux4/3
  Constant7/1 -> Reinterpret/1
  Constant6/1 -> Reinterpret1/1
  Constant5/1 -> Reinterpret2/1
  Constant4/1 -> Reinterpret3/1
  Reinterpret/1 -> Concat2/1
  Reinterpret1/1 -> Concat2/2
  Reinterpret2/1 -> Concat2/3
  Reinterpret3/1 -> Concat2/4
  Constant1/1 -> tv1/1
  Constant2/1 -> tv2/1
  Constant12/1 -> tv7/1
  Constant11/1 -> tv6/1
  Constant10/1 -> tv5/1
  Constant9/1 -> tv4/1
  Constant8/1 -> tv3/1
  Delay9/1 -> valid_out/1
  valid_in/1 -> Mux1/2
  Mux1/1 -> Delay1/1
  [use_tvg] -> Mux1/1
  Constant13/1 -> Mux1/3
  Delay1/1 -> Delay3/1

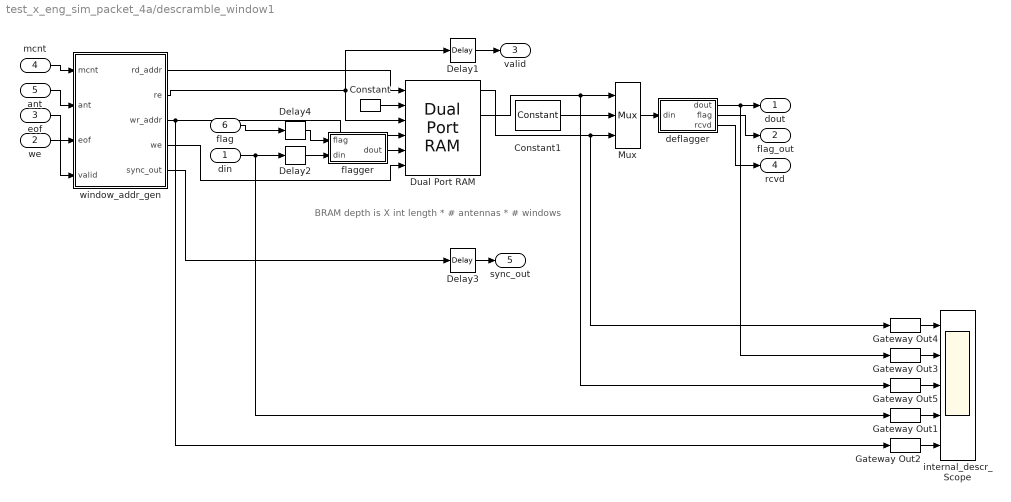
== system test_x_eng_sim_packet_4a/descramble_window1 ==
  note: BRAM depth is
      | X int length * # antennas * # windows
  din : Inport  Port=1  LatchInput=off
  we : Inport  Port=2  LatchInput=off
  eof : Inport  Port=3  LatchInput=off
  mcnt : Inport  Port=4  LatchInput=off
  ant : Inport  Port=5  LatchInput=off
  flag : Inport  Port=6  LatchInput=off
  Constant : xbsIndex_r3/Constant  const=0  equ=P=C  arith_type=Unsigned  n_bits=18  bin_pt=0  opselect=C  inp2=PCIN>>17  opr=+  inp1=P  carry=CIN  iostate=0  explicit_period=on  period=1  dbl_ovrd=off
  Constant1 : xbsIndex_r3/Constant  const=0  equ=P=C  arith_type=Unsigned  n_bits=1  bin_pt=0  opselect=C  inp2=PCIN>>17  opr=+  inp1=P  carry=CIN  iostate=0  explicit_period=off  period=1  dbl_ovrd=off
  Delay1 : xbsIndex_r3/Delay  latency=2  reg_retiming=off  explicit_period=off  period=1  en=off  accept_only_valid=off  init_zero=on  dbl_ovrd=off  show_param=off
      settings: xl_area=[0, 0, 0, 0, 0, 0, 0]
  Delay2 : xbsIndex_r3/Delay  latency=4  reg_retiming=off  explicit_period=off  period=1  en=off  accept_only_valid=off  init_zero=on  dbl_ovrd=off  show_param=off
      settings: xl_area=[0, 0, 0, 0, 0, 0, 0]
  Delay3 : xbsIndex_r3/Delay  latency=2  reg_retiming=off  explicit_period=off  period=1  en=off  accept_only_valid=off  init_zero=on  dbl_ovrd=off  show_param=off
      settings: xl_area=[0, 0, 0, 0, 0, 0, 0]
  Delay4 : xbsIndex_r3/Delay  latency=4  reg_retiming=off  explicit_period=off  period=1  en=off  accept_only_valid=off  init_zero=on  dbl_ovrd=off  show_param=off
      settings: xl_area=[0, 0, 0, 0, 0, 0, 0]
  Dual Port RAM : xbsIndex_r3/Dual Port RAM  depth=2^x_int_bits * 2^ant_bits * 2^window_bits  initVector=0  write_mode_A=Read Before Write  write_mode_B=Read Before Write  latency=2  mem_collision=on  init_zero=on  explicit_period=off  period=1  dbl_ovrd=off  rst_a=off  init_a=0  rst_b=off  init_b=0  show_param=off  distributed_mem=off  use_rpm=off  gen_core=off
      settings: xl_area=[0, 0, 0, 0, 0, 0, 0]
  Gateway Out{1..5} (5 alike) : xbsIndex_r3/Gateway Out  output_type=Double  nbits=8  bin_pt=6  arith_type=Boolean  quantization=Truncate  overflow=Wrap  hdl_port=off  timing_constraint=None  locs_specified=off  LOCs={}  needs_fixed_name=off  show_param=off
      settings: xl_area=[0, 0, 0, 0, 0, 0, 0]
  Mux : xbsIndex_r3/Mux  inputs=2  precision=Full  arith_type="Signed  (2's comp)"  n_bits=8  bin_pt=2  quantization=Truncate  overflow=Wrap  latency=0  explicit_period=off  period=1  en=off  dbl_ovrd=off  show_param=off  mux_type=off  use_rpm=off  gen_core=off
      settings: xl_area=[0, 0, 0, 0, 0, 0, 0]
  deflagger : Subsystem
  flagger : Subsystem
  internal_descr_Scope : Scope  NumInputPorts=5
      settings: TimeRange=1  YMin=-1~-1~0.95~-5~-5  YMax=1~1~1.05~5~5  SaveName=ScopeData11
  window_addr_gen : Subsystem
  dout : Outport
  flag_out : Outport  Port=2
  valid : Outport  Port=3
  rcvd : Outport  Port=4
  sync_out : Outport  Port=5
  wires:
  window_addr_gen/4(we) -> Dual Port RAM/6
  window_addr_gen/3(wr_addr) -> Dual Port RAM/4, Gateway Out2/1
  window_addr_gen/2(re) -> Dual Port RAM/3, Delay1/1
  window_addr_gen/1(rd_addr) -> Dual Port RAM/1
  flagger/1(dout) -> Dual Port RAM/5
  Constant/1 -> Dual Port RAM/2
  Delay1/1 -> valid/1
  we/1 -> window_addr_gen/4(valid)
  eof/1 -> window_addr_gen/3(eof)
  ant/1 -> window_addr_gen/2(ant)
  mcnt/1 -> window_addr_gen/1(mcnt)
  Delay3/1 -> sync_out/1
  window_addr_gen/5(sync_out) -> Delay3/1
  flag/1 -> Delay4/1
  Delay4/1 -> flagger/1(flag)
  din/1 -> Delay2/1, Gateway Out1/1
  Delay2/1 -> flagger/2(din)
  deflagger/3(rcvd) -> rcvd/1
  deflagger/2(flag) -> flag_out/1
  deflagger/1(dout) -> dout/1, Gateway Out3/1
  Dual Port RAM/1 -> Mux/3, Gateway Out4/1
  Mux/1 -> deflagger/1(din)
  Constant1/1 -> Mux/2
  Dual Port RAM/2 -> Mux/1, Gateway Out5/1
  Gateway Out3/1 -> internal_descr_Scope/2
  Gateway Out4/1 -> internal_descr_Scope/1
  Gateway Out5/1 -> internal_descr_Scope/3
  Gateway Out1/1 -> internal_descr_Scope/4
  Gateway Out2/1 -> internal_descr_Scope/5

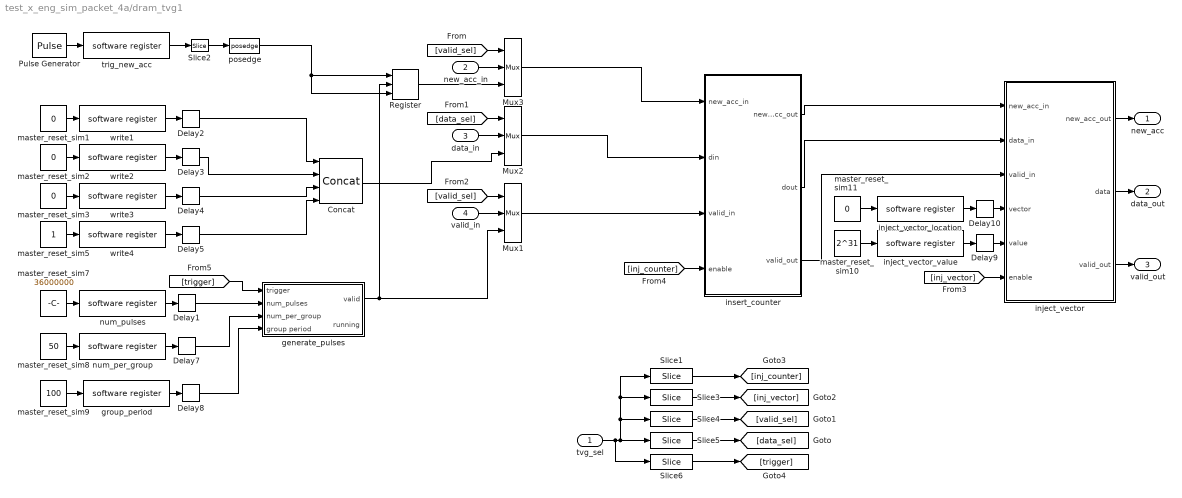
== system test_x_eng_sim_packet_4a/dram_tvg1 ==
  tvg_sel : Inport  Port=1  LatchInput=off
  new_acc_in : Inport  Port=2  LatchInput=off
  data_in : Inport  Port=3  LatchInput=off
  valid_in : Inport  Port=4  LatchInput=off
  Concat : xbsIndex_r3/Concat  num_inputs=4  explicit_period=on  period=1  dbl_ovrd=off
  Delay{1..5,7..10} (9 alike) : xbsIndex_r3/Delay  latency=5  reg_retiming=off  explicit_period=off  period=1  en=off  accept_only_valid=off  init_zero=on  dbl_ovrd=off  show_param=off
      settings: xl_area=[0, 0, 0, 0, 0, 0, 0]
  Mux1 : xbsIndex_r3/Mux  inputs=2  precision=Full  arith_type="Signed  (2's comp)"  n_bits=8  bin_pt=2  quantization=Truncate  overflow=Wrap  latency=0  explicit_period=off  period=1  en=off  dbl_ovrd=off  show_param=off  mux_type=off  use_rpm=off  gen_core=off
      settings: xl_area=[0, 0, 0, 0, 0, 0, 0]
  Mux2 : xbsIndex_r3/Mux  inputs=2  precision=Full  arith_type="Signed  (2's comp)"  n_bits=8  bin_pt=2  quantization=Truncate  overflow=Wrap  latency=0  explicit_period=off  period=1  en=off  dbl_ovrd=off  show_param=off  mux_type=off  use_rpm=off  gen_core=off
      settings: xl_area=[0, 0, 0, 0, 0, 0, 0]
  Mux3 : xbsIndex_r3/Mux  inputs=2  precision=Full  arith_type="Signed  (2's comp)"  n_bits=8  bin_pt=2  quantization=Truncate  overflow=Wrap  latency=0  explicit_period=off  period=1  en=off  dbl_ovrd=off  show_param=off  mux_type=off  use_rpm=off  gen_core=off
      settings: xl_area=[0, 0, 0, 0, 0, 0, 0]
  Pulse Generator : DiscretePulseGenerator  Period=29985  PhaseDelay=600
  Register : xbsIndex_r3/Register  init=0  reg_only_valid=off  explicit_period=off  period=1  rst=on  en=on  out_en=off  dbl_ovrd=off  show_param=off
      settings: xl_area=[0, 0, 0, 0, 0, 0, 0]
  Slice1 : xbsIndex_r3/Slice  mode=Lower Bit Location + Width  nbits=1  bit1=0  base1=MSB of Input  bit0=4  base0=LSB of Input  boolean_output=on  explicit_period=off  period=1  dbl_ovrd=off
  Slice2 : xbsIndex_r3/Slice  mode=Lower Bit Location + Width  nbits=1  bit1=3  base1=LSB of Input  bit0=0  base0=LSB of Input  boolean_output=on  explicit_period=on  period=1  dbl_ovrd=off
  Slice3 : xbsIndex_r3/Slice  mode=Lower Bit Location + Width  nbits=1  bit1=0  base1=MSB of Input  bit0=3  base0=LSB of Input  boolean_output=on  explicit_period=off  period=1  dbl_ovrd=off
  Slice4 : xbsIndex_r3/Slice  mode=Lower Bit Location + Width  nbits=1  bit1=0  base1=MSB of Input  bit0=2  base0=LSB of Input  boolean_output=on  explicit_period=off  period=1  dbl_ovrd=off
  Slice5 : xbsIndex_r3/Slice  mode=Lower Bit Location + Width  nbits=1  bit1=0  base1=MSB of Input  bit0=1  base0=LSB of Input  boolean_output=on  explicit_period=off  period=1  dbl_ovrd=off
  Slice6 : xbsIndex_r3/Slice  mode=Lower Bit Location + Width  nbits=1  bit1=0  base1=MSB of Input  bit0=0  base0=LSB of Input  boolean_output=on  explicit_period=off  period=1  dbl_ovrd=off
  generate_pulses : Subsystem
  group_period : xps_library/software register  Tag=xps:sw_reg  io_dir=From Processor  arith_type=Unsigned  bitwidth=32  bin_pt=0  sample_period=1  gw_name=test_x_eng_sim_packet_4a_dram_tvg1_group_period_user_data_out
  inject_vector : Subsystem  mask{num_vectors=len}
      mask prompts: num_vectors "number of vectors"
  inject_vector_location : xps_library/software register  Tag=xps:sw_reg  io_dir=From Processor  arith_type=Unsigned  bitwidth=32  bin_pt=0  sample_period=1  gw_name=test_x_eng_sim_packet_4a_dram_tvg1_inject_vector_location_user_data_out
  inject_vector_value : xps_library/software register  Tag=xps:sw_reg  io_dir=From Processor  arith_type=Unsigned  bitwidth=32  bin_pt=0  sample_period=1  gw_name=test_x_eng_sim_packet_4a_dram_tvg1_inject_vector_value_user_data_out
  insert_counter : Subsystem  mask{vec_len=len}
      mask prompts: vec_len "Vector Length?"
  master_reset_sim{1..3,11} (4 alike) : Constant  Value=0
  master_reset_sim10 : Constant  Value=2^31
  master_reset_sim5 : Constant
  master_reset_sim7 : Constant  Value=36000000
  master_reset_sim8 : Constant  Value=50
  master_reset_sim9 : Constant  Value=100
  num_per_group : xps_library/software register  Tag=xps:sw_reg  io_dir=From Processor  arith_type=Unsigned  bitwidth=32  bin_pt=0  sample_period=1  gw_name=test_x_eng_sim_packet_4a_dram_tvg1_num_per_group_user_data_out
  num_pulses : xps_library/software register  Tag=xps:sw_reg  io_dir=From Processor  arith_type=Unsigned  bitwidth=32  bin_pt=0  sample_period=1  gw_name=test_x_eng_sim_packet_4a_dram_tvg1_num_pulses_user_data_out
  posedge : casper_library/Misc/posedge  Tag=Rising Edge Detector
  trig_new_acc : xps_library/software register  Tag=xps:sw_reg  io_dir=From Processor  arith_type=Unsigned  bitwidth=32  bin_pt=0  sample_period=1  gw_name=test_x_eng_sim_packet_4a_dram_tvg1_trig_new_acc_user_data_out
  write1 : xps_library/software register  Tag=xps:sw_reg  io_dir=From Processor  arith_type=Unsigned  bitwidth=32  bin_pt=0  sample_period=1  gw_name=test_x_eng_sim_packet_4a_dram_tvg1_write1_user_data_out
  write2 : xps_library/software register  Tag=xps:sw_reg  io_dir=From Processor  arith_type=Unsigned  bitwidth=32  bin_pt=0  sample_period=1  gw_name=test_x_eng_sim_packet_4a_dram_tvg1_write2_user_data_out
  write3 : xps_library/software register  Tag=xps:sw_reg  io_dir=From Processor  arith_type=Unsigned  bitwidth=32  bin_pt=0  sample_period=1  gw_name=test_x_eng_sim_packet_4a_dram_tvg1_write3_user_data_out
  write4 : xps_library/software register  Tag=xps:sw_reg  io_dir=From Processor  arith_type=Unsigned  bitwidth=32  bin_pt=0  sample_period=1  gw_name=test_x_eng_sim_packet_4a_dram_tvg1_write4_user_data_out
  new_acc : Outport
  data_out : Outport  Port=2
  valid_out : Outport  Port=3
  wires:
  trig_new_acc/1 -> Slice2/1
  Pulse Generator/1 -> trig_new_acc/1
  write1/1 -> Delay2/1
  master_reset_sim1/1 -> write1/1
  write2/1 -> Delay3/1
  master_reset_sim2/1 -> write2/1
  write3/1 -> Delay4/1
  master_reset_sim3/1 -> write3/1
  write4/1 -> Delay5/1
  master_reset_sim5/1 -> write4/1
  Delay2/1 -> Concat/1
  Delay3/1 -> Concat/2
  Delay4/1 -> Concat/3
  Delay5/1 -> Concat/4
  Slice2/1 -> posedge/1
  num_pulses/1 -> Delay1/1
  master_reset_sim7/1 -> num_pulses/1
  Delay1/1 -> generate_pulses/2(num_pulses)
  num_per_group/1 -> Delay7/1
  master_reset_sim8/1 -> num_per_group/1
  Delay7/1 -> generate_pulses/3(num_per_group)
  group_period/1 -> Delay8/1
  master_reset_sim9/1 -> group_period/1
  Delay8/1 -> generate_pulses/4(group period)
  Mux1/1 -> insert_counter/3(valid_in)
  valid_in/1 -> Mux1/2
  inject_vector/1(new_acc_out) -> new_acc/1
  inject_vector/2(data) -> data_out/1
  inject_vector/3(valid_out) -> valid_out/1
  insert_counter/1(new_acc_out) -> inject_vector/1(new_acc_in)
  Mux2/1 -> insert_counter/2(din)
  data_in/1 -> Mux2/2
  new_acc_in/1 -> Mux3/2
  Mux3/1 -> insert_counter/1(new_acc_in)
  Slice5/1 -> [data_sel]
  tvg_sel/1 -> Slice5/1, Slice3/1, Slice1/1, Slice4/1, Slice6/1
  Slice4/1 -> [valid_sel]
  [valid_sel] -> Mux3/1
  [data_sel] -> Mux2/1
  [valid_sel] -> Mux1/1
  Slice3/1 -> [inj_vector]
  Slice1/1 -> [inj_counter]
  [trigger] -> generate_pulses/1(trigger)
  insert_counter/2(dout) -> inject_vector/2(data_in)
  insert_counter/3(valid_out) -> inject_vector/3(valid_in)
  Concat/1 -> Mux2/3
  generate_pulses/1(valid) -> Mux1/3, Register/2
  Register/1 -> Mux3/3
  posedge/1 -> Register/1, Register/3
  [inj_vector] -> inject_vector/6(enable)
  Delay10/1 -> inject_vector/4(vector)
  master_reset_sim11/1 -> inject_vector_location/1
  inject_vector_location/1 -> Delay10/1
  Delay9/1 -> inject_vector/5(value)
  master_reset_sim10/1 -> inject_vector_value/1
  inject_vector_value/1 -> Delay9/1
  [inj_counter] -> insert_counter/4(enable)
  Slice6/1 -> [trigger]

== system test_x_eng_sim_packet_4a/fmt_for_dram1 ==
  din : Inport  Port=1  LatchInput=off
  we : Inport  Port=2  LatchInput=off
  sync : Inport  Port=3  LatchInput=off
  Delay1 : xbsIndex_r3/Delay  latency=1  reg_retiming=off  explicit_period=off  period=1  en=off  accept_only_valid=off  init_zero=on  dbl_ovrd=off  show_param=off
      settings: xl_area=[0, 0, 0, 0, 0, 0, 0]
  Delay2 : xbsIndex_r3/Delay  latency=2  reg_retiming=off  explicit_period=off  period=1  en=off  accept_only_valid=off  init_zero=on  dbl_ovrd=off  show_param=off
      settings: xl_area=[0, 0, 0, 0, 0, 0, 0]
  Delay3 : xbsIndex_r3/Delay  latency=1  reg_retiming=off  explicit_period=off  period=1  en=off  accept_only_valid=off  init_zero=on  dbl_ovrd=off  show_param=off
      settings: xl_area=[0, 0, 0, 0, 0, 0, 0]
  Logical4 : xbsIndex_r3/Logical  logical_function=OR  inputs=2  precision=Full  arith_type=Unsigned  n_bits=8  bin_pt=2  align_bp=on  latency=1  explicit_period=off  period=1  en=off  dbl_ovrd=off  show_param=off
      settings: xl_area=[0, 0, 0, 0, 0, 0, 0]
  Mux : xbsIndex_r3/Mux  inputs=2  precision=Full  arith_type="Signed  (2's comp)"  n_bits=8  bin_pt=2  quantization=Truncate  overflow=Wrap  latency=1  explicit_period=off  period=1  en=off  dbl_ovrd=off  show_param=off  mux_type=off  use_rpm=off  gen_core=off
      settings: xl_area=[0, 0, 0, 0, 0, 0, 0]
  Register4 : xbsIndex_r3/Register  init=0  reg_only_valid=off  explicit_period=off  period=1  rst=off  en=on  out_en=off  dbl_ovrd=off  show_param=off
      settings: xl_area=[0, 0, 0, 0, 0, 0, 0]
  mk_4x32bit : Subsystem
  stokes12 : xbsIndex_r3/Slice  mode=Lower Bit Location + Width  nbits=4 * (2*x_n_bits+1+x_int_bits)  bit1=0  base1=MSB of Input  bit0=4 * (2*x_n_bits+1+x_int_bits)  base0=LSB of Input  boolean_output=off  explicit_period=off  period=1  dbl_ovrd=off
  stokes34 : xbsIndex_r3/Slice  mode=Lower Bit Location + Width  nbits=4 * (2*x_n_bits+1+x_int_bits)  bit1=0  base1=MSB of Input  bit0=0  base0=LSB of Input  boolean_output=off  explicit_period=off  period=1  dbl_ovrd=off
  sync_out : Outport
  dout : Outport  Port=2
  valid : Outport  Port=3
  wires:
  Delay2/1 -> sync_out/1
  Logical4/1 -> valid/1
  mk_4x32bit/1(dout) -> dout/1
  Mux/1 -> mk_4x32bit/1(din)
  stokes12/1 -> Mux/2
  stokes34/1 -> Mux/3
  Delay1/1 -> Logical4/1
  we/1 -> Register4/2, Delay3/1
  sync/1 -> Delay2/1
  Register4/1 -> stokes12/1, stokes34/1
  din/1 -> Register4/1
  Delay3/1 -> Logical4/2, Delay1/1, Mux/1
